simulink model "ACDCMG_woPV"  (R2022a)
settings: Solver=FixedStepAuto  StartTime=0.0  StopTime=0.2  FixedStep=Ts  MaxStep=1e-2  RelTol=1e-3
InitFcn:
  | Set_parameters_R2018
values from neighbouring files (symbols this model uses):
  D_invs = 0.05    [Set_parameters_R2018.m]
  dis11 = 3    [Set_parameters_R2018.m]
  dis14 = 2    [Set_parameters_R2018.m]
  dis2 = 0.2    [Set_parameters_R2018.m]
  dis3 = 0.15    [Set_parameters_R2018.m]
  dis4 = 0.4    [Set_parameters_R2018.m]
  dis5 = 0.4    [Set_parameters_R2018.m]
  dis6 = 0.4    [Set_parameters_R2018.m]
  dis8 = 2    [Set_parameters_R2018.m]
  Fnom = 60    [Set_parameters_R2018.m]
  H_invs = 6    [Set_parameters_R2018.m]
  max_min = 1    [Set_parameters_R2018.m]
  P_Load_3 = S_Load_3* PF_Load_3    (= 25500)    [Set_parameters_R2018.m]
  P_nom_inv = 3e3    (= 3000)    [Set_parameters_R2018.m]
  Pnom_T1 = 1.5e6    (= 1500000)    [Set_parameters_R2018.m]
  Pnom_T2 = 1.5e6    (= 1500000)    [Set_parameters_R2018.m]
  Pnom_T3 = 4e6    (= 4000000)    [Set_parameters_R2018.m]
  Ql_Load_3 = S_Load_3 * sin(acos(PF_Load_3))    [Set_parameters_R2018.m]
  R_Load_9 = (Vnom_prim * 1.35)^2 / P_Load_9    (= 1084.6153125)    [Set_parameters_R2018.m]
  R_Load_DC = Vnom_DC^2/ P_Load_DC    (= 45)    [Set_parameters_R2018.m]
  Rl = 0.394    [Set_parameters_R2018.m]
  Rls = 0.198    [Set_parameters_R2018.m]
  Ts = Ts_Power    (= 6.94444444444e-06)    [Set_parameters_R2018.m]
  Ts_Control = 6*Ts_Power    (= 4.16666666667e-05)    [Set_parameters_R2018.m]
  Ts_Power = 1/(24*Fnom)/100    (= 6.94444444444e-06)    [Set_parameters_R2018.m]
  V1_LL_T3 = 69e3    (= 69000)    [Set_parameters_R2018.m]
  Vnom_DC = 300    [Set_parameters_R2018.m]
  Vnom_Diesel = 2.4e3    (= 2400)    [Set_parameters_R2018.m]
  Vnom_prim = 13.8e3    (= 13800)    [Set_parameters_R2018.m]
  Vnom_sec = 220    [Set_parameters_R2018.m]
  Vnom_ter_AC_DC = 150    [Set_parameters_R2018.m]
  Xl = 0.1168    [Set_parameters_R2018.m]
  Xls = 0.1089    [Set_parameters_R2018.m]
undefined symbols (not defined in the file or in its folder): D1, Delta, DiscIntNeverNeededParam, ee_sli_rtmsupport, fn, gcbh, Ion, Lithium, S, sigbuilder_block, VnInv
libraries: powerlib_extras x55, spsCurrentMeasurementLib x53, powerlib_meascontrol x42, spsSeriesRLCBranchLib x32, spsVoltageMeasurementLib x31, spsRMSLib x29, spsThreePhaseVIMeasurementLib x24, simulink x21, spsThreePhaseSeriesRLCBranchLib x19, spsPower3phInstantaneousLib x15, spsPowerLib x12, spsGroundLib x11
(part 7 of 9)

== system ACDCMG_woPV/Grid Bi-directional Converter 1.2 300 (DC) // 150 V (AC) P_nom 3kW1/Power Measurement (Three-Phase)/Continuous ==
  V : Inport
  I : Inport  Port=2
  Complex to Real-Imag : ComplexToRealImag
  Demux2 : Demux  Outputs=3
  Demux3 : Demux  Outputs=3
  Gain1 : Gain  Gain=3/2
  Gain2 : Gain  Gain=3/2
  Gain3 : Gain  Gain=3/2
  Math Function : Math  Operator=conj  SignedPower=on
  Math Function1 : Math  Operator=conj  SignedPower=on
  Math Function2 : Math  Operator=conj  SignedPower=on
  Multiport Switch : MultiPortSwitch  SaturateOnIntegerOverflow=off  InputSameDT=off
  Mux : Mux  Inputs=3
  Mux1 : Mux  Inputs=3
  Negative I2 : Subsystem
  Negative V2 : Subsystem
  Phase-A I : Subsystem
  Phase-A V : Subsystem
  Phase-B I : Subsystem
  Phase-B V : Subsystem
  Phase-C I : Subsystem
  Phase-C V : Subsystem
  Positive I1 : Subsystem
  Positive V1 : Subsystem
  Product1 : Product
  Product2 : Product
  Product3 : Product
  Sequence : Constant  Value=S
  SinCos : Subsystem
  Zero I0 : Subsystem
  Zero V0 : Subsystem
  P : Outport  VectorParamsAs1DForOutWhenUnconnected=off
  Q : Outport  Port=2  VectorParamsAs1DForOutWhenUnconnected=off
  wires:
  Product3/1 -> Gain2/1
  V/1 -> Demux2/1
  Demux2/1 -> Phase-A V/1(Input)
  Demux2/2 -> Phase-B V/1(Input)
  Demux2/3 -> Phase-C V/1(Input)
  Demux3/3 -> Phase-C I/1(Input)
  Demux3/2 -> Phase-B I/1(Input)
  Demux3/1 -> Phase-A I/1(Input)
  I/1 -> Demux3/1
  SinCos/1(SinCos) -> Phase-C I/2(SinCos), Phase-B I/2(SinCos), Phase-A I/2(SinCos), Phase-C V/2(SinCos), Phase-B V/2(SinCos), Phase-A V/2(SinCos)
  Positive I1/1(I1) -> Math Function/1
  Math Function/1 -> Product3/2
  Phase-A V/1(Phasor) -> Mux/1
  Phase-B V/1(Phasor) -> Mux/2
  Phase-C V/1(Phasor) -> Mux/3
  Mux/1 -> Zero V0/1(Phasor_ABC), Negative V2/1(Phasor_ABC), Positive V1/1(Phasor_ABC)
  Phase-A I/1(Phasor) -> Mux1/1
  Phase-B I/1(Phasor) -> Mux1/2
  Phase-C I/1(Phasor) -> Mux1/3
  Mux1/1 -> Positive I1/1(Phasor_ABC), Negative I2/1(Phasor_ABC), Zero I0/1(Phasor_ABC)
  Positive V1/1(V1) -> Product3/1
  Negative I2/1(I2) -> Math Function1/1
  Zero I0/1(I0) -> Math Function2/1
  Product1/1 -> Gain1/1
  Negative V2/1(V2) -> Product1/1
  Math Function1/1 -> Product1/2
  Product2/1 -> Gain3/1
  Zero V0/1(V0) -> Product2/1
  Math Function2/1 -> Product2/2
  Gain2/1 -> Multiport Switch/2
  Gain1/1 -> Multiport Switch/3
  Gain3/1 -> Multiport Switch/4
  Sequence/1 -> Multiport Switch/1
  Multiport Switch/1 -> Complex to Real-Imag/1
  Complex to Real-Imag/1 -> P/1
  Complex to Real-Imag/2 -> Q/1

== system ACDCMG_woPV/Grid Bi-directional Converter 1.2 300 (DC) // 150 V (AC) P_nom 3kW1/Power Measurement (Three-Phase)/Discrete ==
  V : Inport
  I : Inport  Port=2
  Complex to Real-Imag : ComplexToRealImag
  Demux2 : Demux  Outputs=3
  Demux3 : Demux  Outputs=3
  Gain1 : Gain  Gain=3/2
  Gain2 : Gain  Gain=3/2
  Gain3 : Gain  Gain=3/2
  Math Function : Math  Operator=conj  SignedPower=on
  Math Function1 : Math  Operator=conj  SignedPower=on
  Math Function2 : Math  Operator=conj  SignedPower=on
  Multiport Switch : MultiPortSwitch  SaturateOnIntegerOverflow=off  InputSameDT=off
  Mux : Mux  Inputs=3
  Mux1 : Mux  Inputs=3
  Negative I2 : Subsystem
  Negative V2 : Subsystem
  Phase-A I : Subsystem
  Phase-A V : Subsystem
  Phase-B I : Subsystem
  Phase-B V : Subsystem
  Phase-C I : Subsystem
  Phase-C V : Subsystem
  Positive I1 : Subsystem
  Positive V1 : Subsystem
  Product1 : Product
  Product2 : Product
  Product3 : Product
  Sequence : Constant  Value=S
  SinCos : Subsystem
  Zero I0 : Subsystem
  Zero V0 : Subsystem
  P : Outport  VectorParamsAs1DForOutWhenUnconnected=off
  Q : Outport  Port=2  VectorParamsAs1DForOutWhenUnconnected=off
  wires:
  Complex to Real-Imag/2 -> Q/1
  Complex to Real-Imag/1 -> P/1
  Multiport Switch/1 -> Complex to Real-Imag/1
  Sequence/1 -> Multiport Switch/1
  Gain3/1 -> Multiport Switch/4
  Gain1/1 -> Multiport Switch/3
  Gain2/1 -> Multiport Switch/2
  Math Function2/1 -> Product2/2
  Zero V0/1(V0) -> Product2/1
  Product2/1 -> Gain3/1
  Math Function1/1 -> Product1/2
  Negative V2/1(V2) -> Product1/1
  Product1/1 -> Gain1/1
  Zero I0/1(I0) -> Math Function2/1
  Negative I2/1(I2) -> Math Function1/1
  Positive V1/1(V1) -> Product3/1
  Mux1/1 -> Zero I0/1(Phasor_ABC), Negative I2/1(Phasor_ABC), Positive I1/1(Phasor_ABC)
  Phase-C I/1(Phasor) -> Mux1/3
  Phase-B I/1(Phasor) -> Mux1/2
  Phase-A I/1(Phasor) -> Mux1/1
  Mux/1 -> Positive V1/1(Phasor_ABC), Negative V2/1(Phasor_ABC), Zero V0/1(Phasor_ABC)
  Phase-C V/1(Phasor) -> Mux/3
  Phase-B V/1(Phasor) -> Mux/2
  Phase-A V/1(Phasor) -> Mux/1
  Math Function/1 -> Product3/2
  Positive I1/1(I1) -> Math Function/1
  SinCos/1(SinCos) -> Phase-A V/2(SinCos), Phase-B V/2(SinCos), Phase-C V/2(SinCos), Phase-A I/2(SinCos), Phase-C I/2(SinCos), Phase-B I/2(SinCos)
  I/1 -> Demux3/1
  Demux3/1 -> Phase-A I/1(Input)
  Demux3/2 -> Phase-B I/1(Input)
  Demux3/3 -> Phase-C I/1(Input)
  Demux2/3 -> Phase-C V/1(Input)
  Demux2/2 -> Phase-B V/1(Input)
  Demux2/1 -> Phase-A V/1(Input), SinCos/1(In1)
  V/1 -> Demux2/1
  Product3/1 -> Gain2/1

== system ACDCMG_woPV/Grid Bi-directional Converter 1.2 300 (DC) // 150 V (AC) P_nom 3kW2/Control of Inverter/Discrete PWM Generator1 ==
  note: Pierre Giroux, Gilbert Sybille
      | Power System Laboratory, IREQ
      | Hydro-Quebec
  note: PWM Generator
  Uref : Inport
  BL4 : Logic  Operator=NOT  Inputs=1
  BL5 : Logic  Operator=NOT  Inputs=1
  Constant : Constant  Value=Internal_Phase
  Constant1 : Constant  Value=Internal
  Data Type Conversion : DataTypeConversion  OutDataTypeStr=double
  Data Type Conversion1 : DataTypeConversion  OutDataTypeStr=boolean
  Data Type Conversion2 : DataTypeConversion  OutDataTypeStr=boolean
  Gain : Gain  Gain=2*pi*Freq  SaturateOnIntegerOverflow=on  OutDataTypeStr=Inherit: Same as input  ParamDataTypeStr=Inherit: Same as input
  Gain2 : Gain  Gain=pi/180  SaturateOnIntegerOverflow=on  OutDataTypeStr=Inherit: Same as input  ParamDataTypeStr=Inherit: Same as input
  Gain3 : Gain  Gain=-1  SaturateOnIntegerOverflow=on  OutDataTypeStr=Inherit: Same as input  ParamDataTypeStr=Inherit: Same as input
  Mux : Mux  Inputs=2
  Mux1 : Mux  Inputs=2
  Mux2 : Mux  Inputs=2
  Product : Product  InputSameDT=on  SaturateOnIntegerOverflow=on  OutDataTypeStr=Inherit: Same as first input
  Relational Operator : RelationalOperator
  Relational Operator1 : RelationalOperator
  Select1A : Selector  InputPortWidth=Select1_PortWidth  IndexOptions=Index vector (dialog)  Indices=Select1_Elements  OutputSizes=1
  Select1B : Selector  InputPortWidth=Select1_PortWidth  IndexOptions=Index vector (dialog)  Indices=Select1_Elements  OutputSizes=1
  Select3 : Selector  InputPortWidth=Select3_PortWidth  IndexOptions=Index vector (dialog)  Indices=Select3_Elements  OutputSizes=1
  Sum : Sum  Inputs=+++  InputSameDT=on  SaturateOnIntegerOverflow=on  OutDataTypeStr=Inherit: Same as first input
  Switch : Switch  Criteria=u2 > Threshold  SaturateOnIntegerOverflow=off  InputSameDT=off
  Triangle : simulink/Sources/Repeating Sequence  rep_seq_t=[0 1/Fc/4 3/Fc/4 1/Fc]  rep_seq_y=[0 -1 1 0]
  Trigonometric Function : Trigonometry
  m3 : Constant  Value=Phase
  m4 : Constant  Value=mIndex
  t : DigitalClock  SampleTime=Ts
  Pulses : Outport  VectorParamsAs1DForOutWhenUnconnected=off
  wires:
  Mux2/1 -> Select3/1
  Select1B/1 -> Mux2/2
  Select1A/1 -> Mux2/1
  Mux1/1 -> Select1B/1
  Mux/1 -> Select1A/1
  BL5/1 -> Mux1/2
  BL4/1 -> Mux/2
  Gain3/1 -> Relational Operator1/1
  Triangle/1 -> Relational Operator1/2, Relational Operator/2
  Product/1 -> Switch/1
  Constant1/1 -> Switch/2
  Trigonometric Function/1 -> Product/2
  Sum/1 -> Trigonometric Function/1
  m4/1 -> Product/1
  Constant/1 -> Sum/3
  m3/1 -> Gain2/1
  Gain2/1 -> Sum/2
  Gain/1 -> Sum/1
  t/1 -> Gain/1
  Select3/1 -> Data Type Conversion/1
  Data Type Conversion/1 -> Pulses/1
  Relational Operator/1 -> Data Type Conversion1/1
  Data Type Conversion1/1 -> BL4/1, Mux/1
  Relational Operator1/1 -> Data Type Conversion2/1
  Data Type Conversion2/1 -> BL5/1, Mux1/1
  Switch/1 -> Relational Operator/1, Gain3/1
  Uref/1 -> Switch/3

== system ACDCMG_woPV/Grid Bi-directional Converter 1.2 300 (DC) // 150 V (AC) P_nom 3kW2/Control of Inverter/MI Controller ==
  Vabc : Inport
  DC to AC : Constant  Value=1.2
  Demux : Demux  Commented=on  Outputs=3
  Demux1 : Demux  Outputs=3
  Mux : Mux  Inputs=3
  Mux1 : Mux  Inputs=3
  Mux2 : Mux  Inputs=3
  Product : Product  RndMeth=Zero
  Product1 : Product  RndMeth=Zero
  Product2 : Product  RndMeth=Zero
  Subsystem : Subsystem
  Subsystem1 : Subsystem
  Terminator1 : Terminator  Commented=on
  Terminator2 : Terminator  Commented=on
  Terminator3 : Terminator
  Terminator4 : Terminator
  Terminator5 : Terminator  Commented=on
  Vab1 : powerlib_extras/Discrete Measurements/Discrete  RMS value  Commented=on  Freq=60  Mag_Init=0  Ts=20e-6
      settings: SourceProductBaseCode=PS
  Vab5 : powerlib_extras/Discrete Measurements/Discrete  RMS value  Commented=on  Freq=60  Mag_Init=0  Ts=20e-6
      settings: SourceProductBaseCode=PS
  Vab6 : powerlib_extras/Discrete Measurements/Discrete  RMS value  Commented=on  Freq=60  Mag_Init=0  Ts=20e-6
      settings: SourceProductBaseCode=PS
  Vabc_inv : Outport  VectorParamsAs1DForOutWhenUnconnected=off
  m : Outport  Port=2  VectorParamsAs1DForOutWhenUnconnected=off
  wires:
  Product/1 -> Mux2/1
  Product1/1 -> Mux2/2
  Product2/1 -> Mux2/3
  Mux1/1 -> m/1
  Vabc/1 -> Demux/1
  Demux/1 -> Vab6/1
  Demux/2 -> Vab5/1
  Demux/3 -> Vab1/1
  Demux1/1 -> Product/1, Mux1/1
  Demux1/2 -> Product1/1, Mux1/2
  Demux1/3 -> Product2/1, Mux1/3
  Subsystem/1(Va) -> Product/2
  Subsystem/2(Vb) -> Product1/2
  Subsystem/3(Vc) -> Product2/2
  Mux2/1 -> Vabc_inv/1
  Vab6/1 -> Terminator2/1
  Subsystem1/3(wt) -> Terminator3/1
  Subsystem1/2(sin_cos) -> Subsystem/1(sin_cos)
  Subsystem1/1(Frec) -> Terminator4/1
  DC to AC/1 -> Mux/1, Mux/2, Mux/3
  Mux/1 -> Demux1/1
  Vab5/1 -> Terminator1/1
  Vab1/1 -> Terminator5/1

== system ACDCMG_woPV/Grid Bi-directional Converter 1.2 300 (DC) // 150 V (AC) P_nom 3kW2/Control of Inverter/Positive-Sequence Active & Reactive Power1 ==
  note: Discrete 3-phase Positive-Sequence Active & Reactive Power
  note: Pierre Giroux, Gilbert Sybille
      | Power System Simulation Laboratory
      | IREQ, Hydro-Quebc
  Vabc : Inport  PortDimensions=3
  Iabc : Inport  Port=2  PortDimensions=3
  Deg->Rad : Gain  Gain=pi/180  SaturateOnIntegerOverflow=on  OutDataTypeStr=Inherit: Same as input  ParamDataTypeStr=Inherit: Same as input
  Discrete 3-phase Positive-Sequence Fundamental Value (I) : powerlib_extras/Discrete Measurements/Discrete 3-phase Positive-Sequence Fundamental Value  Freq=Freq  Par_Init=Par_Iinit  Ts=Ts
      settings: SourceProductBaseCode=PS
  Discrete 3-phase Positive-Sequence Fundamental Value (V) : powerlib_extras/Discrete Measurements/Discrete 3-phase Positive-Sequence Fundamental Value  Freq=Freq  Par_Init=Par_Vinit  Ts=Ts
      settings: SourceProductBaseCode=PS
  Gain1 : Gain  Gain=3/2  SaturateOnIntegerOverflow=on  OutDataTypeStr=Inherit: Same as input  ParamDataTypeStr=Inherit: Same as input
  Mag->RMS : Gain  Gain=1/sqrt(2)
  Mux1 : Mux  Inputs=2
  Mux2 : Mux  Inputs=2
  Mux3 : Mux  Inputs=2
  Product : Product  InputSameDT=on  SaturateOnIntegerOverflow=on  OutDataTypeStr=Inherit: Same as first input
  Product1 : Product  InputSameDT=on  SaturateOnIntegerOverflow=on  OutDataTypeStr=Inherit: Same as first input
  Product2 : Product  InputSameDT=on  SaturateOnIntegerOverflow=on  OutDataTypeStr=Inherit: Same as first input
  Sum : Sum  Inputs=+-  InputSameDT=on  SaturateOnIntegerOverflow=on  OutDataTypeStr=Inherit: Same as first input
  Trigonometric Function : Trigonometry
  Trigonometric Function1 : Trigonometry  Operator=cos
  W->kW Var->kvar : Gain  Gain=1/1000
  RMS_V_I : Outport
  P_Q(kW) : Outport  Port=2
  Phase_V_I : Outport  Port=3
  PF : Outport  Port=4
  wires:
  Vabc/1 -> Discrete 3-phase Positive-Sequence Fundamental Value (V)/1
  Iabc/1 -> Discrete 3-phase Positive-Sequence Fundamental Value (I)/1
  Discrete 3-phase Positive-Sequence Fundamental Value (V)/2 -> Sum/1, Mux1/1
  Discrete 3-phase Positive-Sequence Fundamental Value (I)/2 -> Sum/2, Mux1/2
  Sum/1 -> Deg->Rad/1
  Deg->Rad/1 -> Trigonometric Function1/1, Trigonometric Function/1
  Trigonometric Function1/1 -> PF/1, Product/2
  Trigonometric Function/1 -> Product1/1
  Mux2/1 -> Gain1/1
  Product/1 -> Mux2/1
  Product1/1 -> Mux2/2
  Product2/1 -> Product/1, Product1/2
  Discrete 3-phase Positive-Sequence Fundamental Value (V)/1 -> Mux3/1, Product2/1
  Discrete 3-phase Positive-Sequence Fundamental Value (I)/1 -> Mux3/2, Product2/2
  Mux1/1 -> Phase_V_I/1
  Mux3/1 -> Mag->RMS/1
  Mag->RMS/1 -> RMS_V_I/1
  Gain1/1 -> W->kW Var->kvar/1
  W->kW Var->kvar/1 -> P_Q(kW)/1

== system ACDCMG_woPV/Grid Bi-directional Converter 1.2 300 (DC) // 150 V (AC) P_nom 3kW2/Control of Inverter/V//F ==
  e : Inport
  io : Inport  Port=2
  i : Inport  Port=3
  Udc : Inport  Port=4
  Constant : Constant  Value=150*sqrt(2)
  Constant1 : Constant  Value=0
  Subsystem : Subsystem
  UIcontrol : Subsystem
  Pulses : Outport  VectorParamsAs1DForOutWhenUnconnected=off
  wires:
  Constant/1 -> UIcontrol/1(ed_ref)
  Constant1/1 -> UIcontrol/3(eq_ref)
  Udc/1 -> UIcontrol/9(Udc)
  e/1 -> Subsystem/1(e)
  i/1 -> Subsystem/3(i)
  Subsystem/1(ed) -> UIcontrol/2(ed)
  Subsystem/2(eq) -> UIcontrol/4(eq)
  Subsystem/3(iod) -> UIcontrol/5(iod)
  Subsystem/4(ioq) -> UIcontrol/6(ioq)
  Subsystem/8("wt ") -> UIcontrol/8("wt ")
  Subsystem/7(w) -> UIcontrol/7(w)
  Subsystem/5(id) -> UIcontrol/11(id)
  Subsystem/6(iq) -> UIcontrol/10(iq)
  io/1 -> Subsystem/2(io)
  UIcontrol/1(Pulses) -> Pulses/1

== system ACDCMG_woPV/Grid Bi-directional Converter 1.2 300 (DC) // 150 V (AC) P_nom 3kW3/Control of Inverter/Positive-Sequence Active & Reactive Power1 ==
  note: Discrete 3-phase Positive-Sequence Active & Reactive Power
  note: Pierre Giroux, Gilbert Sybille
      | Power System Simulation Laboratory
      | IREQ, Hydro-Quebc
  Vabc : Inport  PortDimensions=3
  Iabc : Inport  Port=2  PortDimensions=3
  Deg->Rad : Gain  Gain=pi/180  SaturateOnIntegerOverflow=on  OutDataTypeStr=Inherit: Same as input  ParamDataTypeStr=Inherit: Same as input
  Discrete 3-phase Positive-Sequence Fundamental Value (I) : powerlib_extras/Discrete Measurements/Discrete 3-phase Positive-Sequence Fundamental Value  Freq=Freq  Par_Init=Par_Iinit  Ts=Ts
      settings: SourceProductBaseCode=PS
  Discrete 3-phase Positive-Sequence Fundamental Value (V) : powerlib_extras/Discrete Measurements/Discrete 3-phase Positive-Sequence Fundamental Value  Freq=Freq  Par_Init=Par_Vinit  Ts=Ts
      settings: SourceProductBaseCode=PS
  Gain1 : Gain  Gain=3/2  SaturateOnIntegerOverflow=on  OutDataTypeStr=Inherit: Same as input  ParamDataTypeStr=Inherit: Same as input
  Mag->RMS : Gain  Gain=1/sqrt(2)
  Mux1 : Mux  Inputs=2
  Mux2 : Mux  Inputs=2
  Mux3 : Mux  Inputs=2
  Product : Product  InputSameDT=on  SaturateOnIntegerOverflow=on  OutDataTypeStr=Inherit: Same as first input
  Product1 : Product  InputSameDT=on  SaturateOnIntegerOverflow=on  OutDataTypeStr=Inherit: Same as first input
  Product2 : Product  InputSameDT=on  SaturateOnIntegerOverflow=on  OutDataTypeStr=Inherit: Same as first input
  Sum : Sum  Inputs=+-  InputSameDT=on  SaturateOnIntegerOverflow=on  OutDataTypeStr=Inherit: Same as first input
  Trigonometric Function : Trigonometry
  Trigonometric Function1 : Trigonometry  Operator=cos
  W->kW Var->kvar : Gain  Gain=1/1000
  RMS_V_I : Outport
  P_Q(kW) : Outport  Port=2
  Phase_V_I : Outport  Port=3
  PF : Outport  Port=4
  wires:
  Vabc/1 -> Discrete 3-phase Positive-Sequence Fundamental Value (V)/1
  Iabc/1 -> Discrete 3-phase Positive-Sequence Fundamental Value (I)/1
  Discrete 3-phase Positive-Sequence Fundamental Value (V)/2 -> Sum/1, Mux1/1
  Discrete 3-phase Positive-Sequence Fundamental Value (I)/2 -> Sum/2, Mux1/2
  Sum/1 -> Deg->Rad/1
  Deg->Rad/1 -> Trigonometric Function1/1, Trigonometric Function/1
  Trigonometric Function1/1 -> PF/1, Product/2
  Trigonometric Function/1 -> Product1/1
  Mux2/1 -> Gain1/1
  Product/1 -> Mux2/1
  Product1/1 -> Mux2/2
  Product2/1 -> Product/1, Product1/2
  Discrete 3-phase Positive-Sequence Fundamental Value (V)/1 -> Mux3/1, Product2/1
  Discrete 3-phase Positive-Sequence Fundamental Value (I)/1 -> Mux3/2, Product2/2
  Mux1/1 -> Phase_V_I/1
  Mux3/1 -> Mag->RMS/1
  Mag->RMS/1 -> RMS_V_I/1
  Gain1/1 -> W->kW Var->kvar/1
  W->kW Var->kvar/1 -> P_Q(kW)/1

== system ACDCMG_woPV/Grid Bi-directional Converter 1.2 300 (DC) // 150 V (AC) P_nom 3kW3/Control of Inverter/V//F ==
  e : Inport
  io : Inport  Port=2
  i : Inport  Port=3
  Udc : Inport  Port=4
  Constant : Constant  Value=150*sqrt(2)
  Constant1 : Constant  Value=0
  Constant2 : Constant  Commented=on
  Constant3 : Constant  Commented=on
  Constant4 : Constant
  From : From  Commented=on  GotoTag=P_mea_inv  TagVisibility=global
  Gain : Gain  Commented=on  Gain=1/P_nom_inv
  Gain1 : Gain  Gain=Fnom
  Gain2 : Gain  Commented=on  Gain=-1
  Scope : Scope  NumInputPorts=2
  Subsystem : Subsystem
  Sum : Sum  Commented=on  Inputs=|+-
  Sum1 : Sum  Commented=on  Inputs=|++
  Transfer Fcn : TransferFcn  Commented=on  Denominator=[2*H_invs D_invs]
  UIcontrol : Subsystem
  wires:
  Constant/1 -> UIcontrol/1(ed_ref)
  Constant1/1 -> UIcontrol/3(eq_ref)
  Udc/1 -> UIcontrol/9(Udc)
  e/1 -> Subsystem/1(e)
  i/1 -> Subsystem/3(i)
  Subsystem/1(ed) -> UIcontrol/2(ed)
  Subsystem/2(eq) -> UIcontrol/4(eq)
  Subsystem/3(iod) -> UIcontrol/5(iod)
  Subsystem/4(ioq) -> UIcontrol/6(ioq)
  Subsystem/8("wt ") -> UIcontrol/8("wt ")
  Subsystem/7(w) -> UIcontrol/7(w)
  Subsystem/5(id) -> UIcontrol/11(id)
  Subsystem/6(iq) -> UIcontrol/10(iq)
  io/1 -> Subsystem/2(io)
  From/1 -> Gain/1
  Gain1/1 -> Scope/1, Subsystem/4(fcmd)
  Gain/1 -> Scope/2, Sum/1
  Constant2/1 -> Sum/2
  Sum/1 -> Gain2/1
  Gain2/1 -> Transfer Fcn/1
  Transfer Fcn/1 -> Sum1/1
  Constant3/1 -> Sum1/2
  Constant4/1 -> Gain1/1

== system ACDCMG_woPV/Inverter 300 (DC) // 150 V (AC) P_nom 3kW4/Control of Inverter/Positive-Sequence Active & Reactive Power1 ==
  note: Discrete 3-phase Positive-Sequence Active & Reactive Power
  note: Pierre Giroux, Gilbert Sybille
      | Power System Simulation Laboratory
      | IREQ, Hydro-Quebc
  Vabc : Inport  PortDimensions=3
  Iabc : Inport  Port=2  PortDimensions=3
  Deg->Rad : Gain  Gain=pi/180  SaturateOnIntegerOverflow=on  OutDataTypeStr=Inherit: Same as input  ParamDataTypeStr=Inherit: Same as input
  Discrete 3-phase Positive-Sequence Fundamental Value (I) : powerlib_extras/Discrete Measurements/Discrete 3-phase Positive-Sequence Fundamental Value  Freq=Freq  Par_Init=Par_Iinit  Ts=Ts
      settings: SourceProductBaseCode=PS
  Discrete 3-phase Positive-Sequence Fundamental Value (V) : powerlib_extras/Discrete Measurements/Discrete 3-phase Positive-Sequence Fundamental Value  Freq=Freq  Par_Init=Par_Vinit  Ts=Ts
      settings: SourceProductBaseCode=PS
  Gain1 : Gain  Gain=3/2  SaturateOnIntegerOverflow=on  OutDataTypeStr=Inherit: Same as input  ParamDataTypeStr=Inherit: Same as input
  Mag->RMS : Gain  Gain=1/sqrt(2)
  Mux1 : Mux  Inputs=2
  Mux2 : Mux  Inputs=2
  Mux3 : Mux  Inputs=2
  Product : Product  InputSameDT=on  SaturateOnIntegerOverflow=on  OutDataTypeStr=Inherit: Same as first input
  Product1 : Product  InputSameDT=on  SaturateOnIntegerOverflow=on  OutDataTypeStr=Inherit: Same as first input
  Product2 : Product  InputSameDT=on  SaturateOnIntegerOverflow=on  OutDataTypeStr=Inherit: Same as first input
  Sum : Sum  Inputs=+-  InputSameDT=on  SaturateOnIntegerOverflow=on  OutDataTypeStr=Inherit: Same as first input
  Trigonometric Function : Trigonometry
  Trigonometric Function1 : Trigonometry  Operator=cos
  W->kW Var->kvar : Gain  Gain=1/1000
  RMS_V_I : Outport
  P_Q(kW) : Outport  Port=2
  Phase_V_I : Outport  Port=3
  PF : Outport  Port=4
  wires:
  Vabc/1 -> Discrete 3-phase Positive-Sequence Fundamental Value (V)/1
  Iabc/1 -> Discrete 3-phase Positive-Sequence Fundamental Value (I)/1
  Discrete 3-phase Positive-Sequence Fundamental Value (V)/2 -> Sum/1, Mux1/1
  Discrete 3-phase Positive-Sequence Fundamental Value (I)/2 -> Sum/2, Mux1/2
  Sum/1 -> Deg->Rad/1
  Deg->Rad/1 -> Trigonometric Function1/1, Trigonometric Function/1
  Trigonometric Function1/1 -> PF/1, Product/2
  Trigonometric Function/1 -> Product1/1
  Mux2/1 -> Gain1/1
  Product/1 -> Mux2/1
  Product1/1 -> Mux2/2
  Product2/1 -> Product/1, Product1/2
  Discrete 3-phase Positive-Sequence Fundamental Value (V)/1 -> Mux3/1, Product2/1
  Discrete 3-phase Positive-Sequence Fundamental Value (I)/1 -> Mux3/2, Product2/2
  Mux1/1 -> Phase_V_I/1
  Mux3/1 -> Mag->RMS/1
  Mag->RMS/1 -> RMS_V_I/1
  Gain1/1 -> W->kW Var->kvar/1
  W->kW Var->kvar/1 -> P_Q(kW)/1

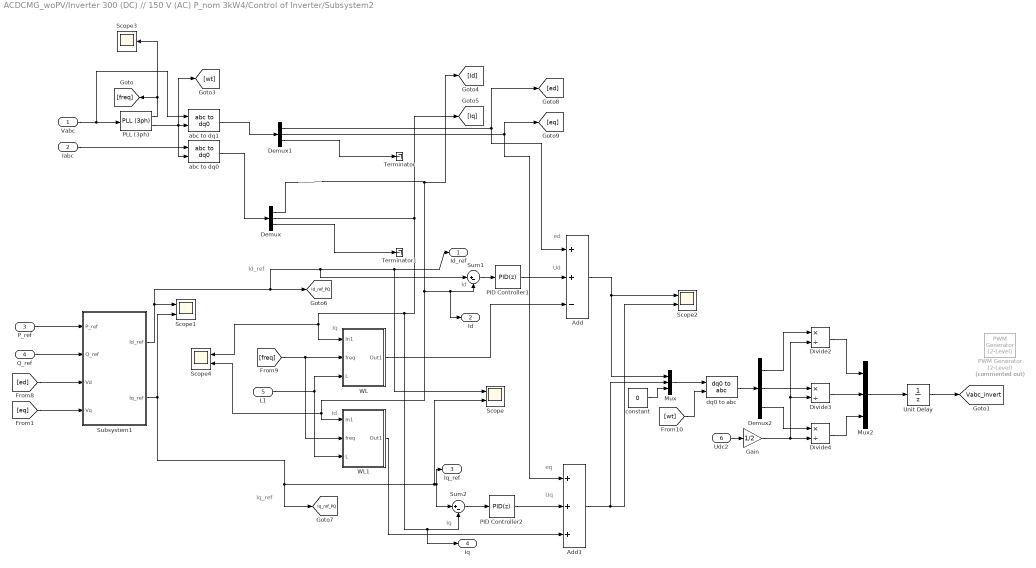
== system ACDCMG_woPV/Inverter 300 (DC) // 150 V (AC) P_nom 3kW4/Control of Inverter/Subsystem2 ==
  note: Iq_ref
  note: Id
  note: Id_ref
  note: Ud
  note: Uq
  note: eq
  note: ed
  note: Iq
  note: Id
  note: Iq
  Vabc : Inport
  Iabc : Inport  Port=2
  P_ref : Inport  Port=3
  Q_ref : Inport  Port=4
  L1 : Inport  Port=5
  Udc2 : Inport  Port=6
  Add : Sum  Inputs=++-
  Add1 : Sum  Inputs=+++
  Demux : Demux  Outputs=3
  Demux1 : Demux  Outputs=3
  Demux2 : Demux  Outputs=3
  Divide2 : Product  Inputs=*/
  Divide3 : Product  Inputs=*/
  Divide4 : Product  Inputs=*/
  Gain : Gain  Gain=1/2
  Mux : Mux  Inputs=3
  Mux2 : Mux  Inputs=3
  PID Controller1 : slpidlib/PID Controller  Controller=PID  Form=Parallel  TimeDomain=Discrete-time  UseExternalTs=off  SampleTime=Ts_Control  IntegratorMethod=Forward Euler  FilterMethod=Forward Euler  ControllerParametersSource=internal  P=Kp  I=Ki  UseKiTs=off  D=Kd  N=100  UseFilter=on  TunerSelectOption=Transfer Function Based (PID Tuner App)  InitialConditionSource=internal  InitialConditionForIntegrator=0  InitialConditionForFilter=0  DifferentiatorICPrevScaledInput=0  ExternalReset=none  TrackingMode=off  Kt=1  LimitOutput=off  SatLimitsSource=internal  UpperSaturationLimit=inf  LowerSaturationLimit=-inf  LinearizeAsGain=on  AntiWindupMode=none  Kb=1  POutMin=[]  POutMax=[]  IOutMin=[]  IOutMax=[]  DOutMin=[]  DOutMax=[]  NOutMin=[]  NOutMax=[]  SumOutMin=[]  SumOutMax=[]  SaturationOutMin=[]  SaturationOutMax=[]  PParamMin=[]  PParamMax=[]  IParamMin=[]  IParamMax=[]  DParamMin=[]  DParamMax=[]  NParamMin=[]  NParamMax=[]  KbParamMin=[]  KbParamMax=[]  KtParamMin=[]  KtParamMax=[]  KbOutMin=[]  KbOutMax=[]  KtOutMin=[]  KtOutMax=[]  IntegratorOutMin=[]  IntegratorOutMax=[]  FilterOutMin=[]  FilterOutMax=[]  SumI1OutMin=[]  SumI1OutMax=[]  SumI2OutMin=[]  SumI2OutMax=[]  SumI3OutMin=[]  SumI3OutMax=[]  SumI4OutMin=[]  SumI4OutMax=[]  SumDOutMin=[]  SumDOutMax=[]  DifferentiatorOutMin=[]  DifferentiatorOutMax=[]  FilterDiffOutCoefMin=[]  FilterDiffOutCoefMax=[]  ReciprocalOutMin=[]  ReciprocalOutMax=[]  SumDenOutMin=[]  SumDenOutMax=[]  SumNumOutMin=[]  SumNumOutMax=[]  DivideOutMin=[]  DivideOutMax=[]  UdiffTsProdOutMin=[]  UdiffTsProdOutMax=[]  NTsProdOutMin=[]  NTsProdOutMax=[]  UintegralTsProdOutMin=[]  UintegralTsProdOutMax=[]  UngainTsProdOutMin=[]  UngainTsProdOutMax=[]  IntegratorContinuousStateAttributes=''  IntegratorStateMustResolveToSignalObject=off  IntegratorRTWStateStorageClass=Auto  FilterContinuousStateAttributes=''  FilterStateMustResolveToSignalObject=off  FilterRTWStateStorageClass=Auto  ParallelPVariant=InternalParameters  IdealPVariant=Disabled  IVariant=InternalParameters  DVariant=InternalParameters  IntegratorVariant=Discrete  SatVariant=Disabled  AWVariant=Passthrough  PCopyVariant=Disabled  TRVariant=Disabled  FdbkBlocksVariant=Forward  IdealPFdbkVariant=Disabled  SatFdbkVariant=Disabled  DerivativeFilterVariant=ForwardEulerFilter  NVariant=InternalParameters  NCopyVariant=Disabled  FilterICVariant=InternalICsFilter  IntegratorICVariant=InternalICs  ExternalResetVariant=Disabled  TRSumVariant=Passthrough  SumFdbkVariant=Disabled  SumVariant=Sum_PID  TsampFilterVariant=InternalTs  TsampNgainVariant=Passthrough  TsampIntegralVariant=Passthrough  ExternalSaturationOutDataTypeStr=Inherit: Same as second input  aMode=0
  PID Controller2 : slpidlib/PID Controller  Controller=PID  Form=Parallel  TimeDomain=Discrete-time  UseExternalTs=off  SampleTime=Ts_Control  IntegratorMethod=Forward Euler  FilterMethod=Forward Euler  ControllerParametersSource=internal  P=Kp  I=Ki  UseKiTs=off  D=Kd  N=100  UseFilter=on  TunerSelectOption=Transfer Function Based (PID Tuner App)  InitialConditionSource=internal  InitialConditionForIntegrator=0  InitialConditionForFilter=0  DifferentiatorICPrevScaledInput=0  ExternalReset=none  TrackingMode=off  Kt=1  LimitOutput=off  SatLimitsSource=internal  UpperSaturationLimit=inf  LowerSaturationLimit=-inf  LinearizeAsGain=on  AntiWindupMode=none  Kb=1  POutMin=[]  POutMax=[]  IOutMin=[]  IOutMax=[]  DOutMin=[]  DOutMax=[]  NOutMin=[]  NOutMax=[]  SumOutMin=[]  SumOutMax=[]  SaturationOutMin=[]  SaturationOutMax=[]  PParamMin=[]  PParamMax=[]  IParamMin=[]  IParamMax=[]  DParamMin=[]  DParamMax=[]  NParamMin=[]  NParamMax=[]  KbParamMin=[]  KbParamMax=[]  KtParamMin=[]  KtParamMax=[]  KbOutMin=[]  KbOutMax=[]  KtOutMin=[]  KtOutMax=[]  IntegratorOutMin=[]  IntegratorOutMax=[]  FilterOutMin=[]  FilterOutMax=[]  SumI1OutMin=[]  SumI1OutMax=[]  SumI2OutMin=[]  SumI2OutMax=[]  SumI3OutMin=[]  SumI3OutMax=[]  SumI4OutMin=[]  SumI4OutMax=[]  SumDOutMin=[]  SumDOutMax=[]  DifferentiatorOutMin=[]  DifferentiatorOutMax=[]  FilterDiffOutCoefMin=[]  FilterDiffOutCoefMax=[]  ReciprocalOutMin=[]  ReciprocalOutMax=[]  SumDenOutMin=[]  SumDenOutMax=[]  SumNumOutMin=[]  SumNumOutMax=[]  DivideOutMin=[]  DivideOutMax=[]  UdiffTsProdOutMin=[]  UdiffTsProdOutMax=[]  NTsProdOutMin=[]  NTsProdOutMax=[]  UintegralTsProdOutMin=[]  UintegralTsProdOutMax=[]  UngainTsProdOutMin=[]  UngainTsProdOutMax=[]  IntegratorContinuousStateAttributes=''  IntegratorStateMustResolveToSignalObject=off  IntegratorRTWStateStorageClass=Auto  FilterContinuousStateAttributes=''  FilterStateMustResolveToSignalObject=off  FilterRTWStateStorageClass=Auto  ParallelPVariant=InternalParameters  IdealPVariant=Disabled  IVariant=InternalParameters  DVariant=InternalParameters  IntegratorVariant=Discrete  SatVariant=Disabled  AWVariant=Passthrough  PCopyVariant=Disabled  TRVariant=Disabled  FdbkBlocksVariant=Forward  IdealPFdbkVariant=Disabled  SatFdbkVariant=Disabled  DerivativeFilterVariant=ForwardEulerFilter  NVariant=InternalParameters  NCopyVariant=Disabled  FilterICVariant=InternalICsFilter  IntegratorICVariant=InternalICs  ExternalResetVariant=Disabled  TRSumVariant=Passthrough  SumFdbkVariant=Disabled  SumVariant=Sum_PID  TsampFilterVariant=InternalTs  TsampNgainVariant=Passthrough  TsampIntegralVariant=Passthrough  ExternalSaturationOutDataTypeStr=Inherit: Same as second input  aMode=0
  PLL (3ph) : spsPLL3phLib/PLL (3ph)  Fmin=59.5  Par_Init=[0, 60]  ParK=[180, 3200, 1]  TcD=1e-4  MaxRateChangeFreq=12  FilterCutOffFreq=25  Ts=Ts_Control  AGC=on
  PWM Generator (2-Level) : spsPWMGenerator2LevelLib/PWM Generator (2-Level)  Commented=on  ModulatorType=Three-phase bridge (6 pulses)  ModulatorMode=Unsynchronized  Fc=15000  Pc=90  nF=27  MinMax="[ -1  1 ]"  SamplingTechnique=Natural  ModulatingSignals=off  m=0.8  Freq=60  Phase=0  Ts=Ts_Power  ShowCarrierOutport=off
  Scope{,1..2,4} (4 alike) : Scope  NumInputPorts=2
  Scope3 : Scope
  Subsystem1 : Subsystem
  Sum1 : Sum  Inputs=|+-
  Sum2 : Sum  Inputs=|+-
  Terminator : Terminator
  Terminator1 : Terminator
  Unit Delay : UnitDelay  SampleTime=-1  HasFrameUpgradeWarning=on
  WL : Subsystem
  WL1 : Subsystem
  abc to dq0 : spsabctodq0Lib/abc to dq0  Alignment=90 degrees behind phase A axis
  abc to dq1 : spsabctodq0Lib/abc to dq0  Alignment=90 degrees behind phase A axis
  constant : Constant  Value=0
  dq0 to abc : spsdq0toabcLib/dq0 to abc  Alignment=90 degrees behind phase A axis
  Id_ref : Outport
  Id : Outport  Port=2
  Iq_ref : Outport  Port=3
  Iq : Outport  Port=4
  tag scope: Id_ref_PQ=global, Iq_ref_PQ=global, Vabc_invert=global
  wires:
  abc to dq1/1 -> Demux1/1
  Sum1/1 -> PID Controller1/1
  Iabc/1 -> abc to dq0/1
  Vabc/1 -> abc to dq1/1, PLL (3ph)/1
  PLL (3ph)/2 -> [wt], abc to dq1/2, abc to dq0/2
  Demux1/1 -> Add/1, [ed]
  L1/1 -> WL/3(L), WL1/3(L)
  WL/1(Out1) -> Add/3
  [freq] -> WL1/2(freq), WL/2(freq)
  PLL (3ph)/1 -> Scope3/1, [freq]
  Demux2/1 -> Divide2/1
  Add/1 -> Mux/1, Scope2/1
  PID Controller2/1 -> Add1/2
  Sum2/1 -> PID Controller2/1
  Demux2/2 -> Divide3/1
  WL1/1(Out1) -> Add1/3
  Demux1/2 -> Add1/1, [eq]
  Add1/1 -> Mux/2, Scope2/2
  Gain/1 -> Divide3/2, Divide2/2, Divide4/2
  Divide4/1 -> Mux2/3
  Divide2/1 -> Mux2/1
  Mux/1 -> dq0 to abc/1
  Demux2/3 -> Divide4/1
  Divide3/1 -> Mux2/2
  dq0 to abc/1 -> Demux2/1
  PID Controller1/1 -> Add/2
  [wt] -> dq0 to abc/2
  Udc2/1 -> Gain/1
  Demux1/3 -> Terminator/1
  Demux/3 -> Terminator1/1
  constant/1 -> Mux/3
  P_ref/1 -> Subsystem1/1(P_ref)
  Q_ref/1 -> Subsystem1/2(Q_ref)
  [ed] -> Subsystem1/3(Vd)
  [eq] -> Subsystem1/4(Vq)
  Subsystem1/2(Iq_ref) -> Scope1/2, [Iq_ref_PQ], Scope/2, Iq_ref/1, Sum2/1
  Subsystem1/1(Id_ref) -> Sum1/1, Scope/1, Id_ref/1, [Id_ref_PQ], Scope1/1
  Demux/1 -> Scope4/2, WL1/1(In1), Id/1, Sum1/2, [Id]
  Demux/2 -> [Iq], Scope4/1, WL/1(In1), Iq/1, Sum2/2
  abc to dq0/1 -> Demux/1
  Mux2/1 -> Unit Delay/1
  Unit Delay/1 -> [Vabc_invert]

== system ACDCMG_woPV/Inverter 300 (DC) // 150 V (AC) P_nom 3kW4/Control of Inverter/V//F ==
  e : Inport
  io : Inport  Port=2
  i : Inport  Port=3
  Udc : Inport  Port=4
  Constant : Constant  Value=150*sqrt(2)
  Constant1 : Constant  Value=0
  Constant2 : Constant  Commented=on
  Constant3 : Constant  Commented=on
  Constant4 : Constant
  From : From  Commented=on  GotoTag=P_mea_inv  TagVisibility=global
  Gain : Gain  Commented=on  Gain=1/P_nom_inv
  Gain1 : Gain  Gain=Fnom
  Gain2 : Gain  Commented=on  Gain=-1
  Scope : Scope  NumInputPorts=2
  Subsystem : Subsystem
  Sum : Sum  Commented=on  Inputs=|+-
  Sum1 : Sum  Commented=on  Inputs=|++
  Transfer Fcn : TransferFcn  Commented=on  Denominator=[2*H_invs D_invs]
  UIcontrol : Subsystem
  wires:
  Constant/1 -> UIcontrol/1(ed_ref)
  Constant1/1 -> UIcontrol/3(eq_ref)
  Udc/1 -> UIcontrol/9(Udc)
  e/1 -> Subsystem/1(e)
  i/1 -> Subsystem/3(i)
  Subsystem/1(ed) -> UIcontrol/2(ed)
  Subsystem/2(eq) -> UIcontrol/4(eq)
  Subsystem/3(iod) -> UIcontrol/5(iod)
  Subsystem/4(ioq) -> UIcontrol/6(ioq)
  Subsystem/8("wt ") -> UIcontrol/8("wt ")
  Subsystem/7(w) -> UIcontrol/7(w)
  Subsystem/5(id) -> UIcontrol/11(id)
  Subsystem/6(iq) -> UIcontrol/10(iq)
  io/1 -> Subsystem/2(io)
  From/1 -> Gain/1
  Gain1/1 -> Scope/1, Subsystem/4(fcmd)
  Gain/1 -> Scope/2, Sum/1
  Constant2/1 -> Sum/2
  Sum/1 -> Gain2/1
  Gain2/1 -> Transfer Fcn/1
  Transfer Fcn/1 -> Sum1/1
  Constant3/1 -> Sum1/2
  Constant4/1 -> Gain1/1

== system ACDCMG_woPV/Grid Bi-directional Converter 1.1 300 (DC) // 150 V (AC) P_nom 3kW/Control of Inverter/MI Controller/OP max // min ==
  note: DC to AC
  note: AC to DC
  Constant2 : Constant  Value=max_min
  OP_max1 : Constant  Value=1.2
  OP_min1 : Constant
  Switch2 : Switch  Criteria=u2 > Threshold  SaturateOnIntegerOverflow=off  InputSameDT=off
  ctrl : Outport  VectorParamsAs1DForOutWhenUnconnected=off
  wires:
  OP_max1/1 -> Switch2/1
  OP_min1/1 -> Switch2/3
  Constant2/1 -> Switch2/2
  Switch2/1 -> ctrl/1

== system ACDCMG_woPV/Grid Bi-directional Converter 1.1 300 (DC) // 150 V (AC) P_nom 3kW/Control of Inverter/MI Controller/Subsystem ==
  sin_cos : Inport  PortDimensions=2
  Demux : Demux  Outputs=2
      settings: DisplayOption=none
  Fcn2 : Fcn  Expr=1*u[1]
  Fcn4 : Fcn  Expr=1*u[3]
  Fcn5 : Fcn  Expr=1*u[5]
  K1 : Constant  Value=0.5
  K2 : Constant  Value=sqrt(3)/2
  Mux2 : Mux  Inputs=6
  Product{,1..3} (4 alike) : Product  InputSameDT=on  SaturateOnIntegerOverflow=on  OutDataTypeStr=Inherit: Same as first input
  Sum : Sum  Inputs=--  InputSameDT=on  SaturateOnIntegerOverflow=on  OutDataTypeStr=Inherit: Same as first input
  Sum1 : Sum  Inputs=-+  InputSameDT=on  SaturateOnIntegerOverflow=on  OutDataTypeStr=Inherit: Same as first input
  Sum2 : Sum  Inputs=--  InputSameDT=on  SaturateOnIntegerOverflow=on  OutDataTypeStr=Inherit: Same as first input
  Sum3 : Sum  Inputs=--  InputSameDT=on  SaturateOnIntegerOverflow=on  OutDataTypeStr=Inherit: Same as first input
  Va : Outport  VectorParamsAs1DForOutWhenUnconnected=off
  Vb : Outport  Port=2  VectorParamsAs1DForOutWhenUnconnected=off
  Vc : Outport  Port=3  VectorParamsAs1DForOutWhenUnconnected=off
  wires:
  sin_cos/1 -> Demux/1
  Demux/1 -> Product/1, Product2/1, Sum2/2, Mux2/1  "sin(wt)"
  Product/1 -> Sum/1
  Product1/1 -> Sum/2
  Product3/1 -> Sum1/1
  Product2/1 -> Sum1/2
  Sum3/1 -> Mux2/6  "cos(wt+2pi/3)"
  Sum2/1 -> Mux2/5  "sin(wt+2pi/3)"
  K1/1 -> Product/2, Product3/2
  K2/1 -> Product1/2, Product2/2
  Sum/1 -> Mux2/3, Sum2/1  "sin(wt-2pi/3)"
  Sum1/1 -> Mux2/4, Sum3/1  "cos(wt-2pi/3)"
  Demux/2 -> Sum3/2, Product3/1, Product1/1, Mux2/2  "cos(wt)"
  Mux2/1 -> Fcn2/1, Fcn4/1, Fcn5/1
  Fcn2/1 -> Va/1
  Fcn4/1 -> Vb/1
  Fcn5/1 -> Vc/1

== system ACDCMG_woPV/Grid Bi-directional Converter 1.1 300 (DC) // 150 V (AC) P_nom 3kW/Control of Inverter/MI Controller/Subsystem1 ==
  note: AC to DC
  note: DC to AC
  Constant1 : Constant  Value=max_min
  Constant2 : Constant  Value=2*pi
  Deg->Rad : Gain  Gain=pi/180  SaturateOnIntegerOverflow=on  OutDataTypeStr=Inherit: Same as input  ParamDataTypeStr=Inherit: Same as input
  Freq1 : Constant  Value=Fnom
  Freq2 : Constant  Value=2*pi
  Math Function : Math  Operator=mod  SignedPower=on
  Mux5 : Mux  Inputs=2
  OP_max1 : Constant  Value=0
  OP_min1 : Constant  Value=228
  Product7 : Product  Inputs=***  InputSameDT=on  SaturateOnIntegerOverflow=on  OutDataTypeStr=Inherit: Same as first input
  Sum : Sum  InputSameDT=on  SaturateOnIntegerOverflow=on  OutDataTypeStr=Inherit: Same as first input
  Switch2 : Switch  Criteria=u2 > Threshold  SaturateOnIntegerOverflow=off  InputSameDT=off
  Trigonometric Function : Trigonometry
  Trigonometric Function1 : Trigonometry  Operator=cos
  t : DigitalClock  SampleTime=Ts
  Frec : Outport  VectorParamsAs1DForOutWhenUnconnected=off
  sin_cos : Outport  Port=2  VectorParamsAs1DForOutWhenUnconnected=off
  wt : Outport  Port=3  VectorParamsAs1DForOutWhenUnconnected=off
  wires:
  Switch2/1 -> Deg->Rad/1
  Deg->Rad/1 -> Sum/2
  Freq1/1 -> Frec/1, Product7/1
  Trigonometric Function/1 -> Mux5/1
  Sum/1 -> Math Function/1
  Trigonometric Function1/1 -> Mux5/2
  Product7/1 -> Sum/1
  Freq2/1 -> Product7/3
  Constant2/1 -> Math Function/2
  t/1 -> Product7/2
  Math Function/1 -> wt/1, Trigonometric Function1/1, Trigonometric Function/1
  Mux5/1 -> sin_cos/1
  Constant1/1 -> Switch2/2
  OP_max1/1 -> Switch2/1
  OP_min1/1 -> Switch2/3

== system ACDCMG_woPV/Grid Bi-directional Converter 1.1 300 (DC) // 150 V (AC) P_nom 3kW1/Control of Inverter/MI Controller/OP max // min ==
  note: DC to AC
  note: AC to DC
  Constant2 : Constant  Value=max_min
  OP_max1 : Constant  Value=1.2
  OP_min1 : Constant
  Switch2 : Switch  Criteria=u2 > Threshold  SaturateOnIntegerOverflow=off  InputSameDT=off
  ctrl : Outport  VectorParamsAs1DForOutWhenUnconnected=off
  wires:
  OP_max1/1 -> Switch2/1
  OP_min1/1 -> Switch2/3
  Constant2/1 -> Switch2/2
  Switch2/1 -> ctrl/1

== system ACDCMG_woPV/Grid Bi-directional Converter 1.1 300 (DC) // 150 V (AC) P_nom 3kW1/Control of Inverter/MI Controller/Subsystem ==
  sin_cos : Inport  PortDimensions=2
  Demux : Demux  Outputs=2
      settings: DisplayOption=none
  Fcn2 : Fcn  Expr=1*u[1]
  Fcn4 : Fcn  Expr=1*u[3]
  Fcn5 : Fcn  Expr=1*u[5]
  K1 : Constant  Value=0.5
  K2 : Constant  Value=sqrt(3)/2
  Mux2 : Mux  Inputs=6
  Product{,1..3} (4 alike) : Product  InputSameDT=on  SaturateOnIntegerOverflow=on  OutDataTypeStr=Inherit: Same as first input
  Sum : Sum  Inputs=--  InputSameDT=on  SaturateOnIntegerOverflow=on  OutDataTypeStr=Inherit: Same as first input
  Sum1 : Sum  Inputs=-+  InputSameDT=on  SaturateOnIntegerOverflow=on  OutDataTypeStr=Inherit: Same as first input
  Sum2 : Sum  Inputs=--  InputSameDT=on  SaturateOnIntegerOverflow=on  OutDataTypeStr=Inherit: Same as first input
  Sum3 : Sum  Inputs=--  InputSameDT=on  SaturateOnIntegerOverflow=on  OutDataTypeStr=Inherit: Same as first input
  Va : Outport  VectorParamsAs1DForOutWhenUnconnected=off
  Vb : Outport  Port=2  VectorParamsAs1DForOutWhenUnconnected=off
  Vc : Outport  Port=3  VectorParamsAs1DForOutWhenUnconnected=off
  wires:
  sin_cos/1 -> Demux/1
  Demux/1 -> Product/1, Product2/1, Sum2/2, Mux2/1  "sin(wt)"
  Product/1 -> Sum/1
  Product1/1 -> Sum/2
  Product3/1 -> Sum1/1
  Product2/1 -> Sum1/2
  Sum3/1 -> Mux2/6  "cos(wt+2pi/3)"
  Sum2/1 -> Mux2/5  "sin(wt+2pi/3)"
  K1/1 -> Product/2, Product3/2
  K2/1 -> Product1/2, Product2/2
  Sum/1 -> Mux2/3, Sum2/1  "sin(wt-2pi/3)"
  Sum1/1 -> Mux2/4, Sum3/1  "cos(wt-2pi/3)"
  Demux/2 -> Sum3/2, Product3/1, Product1/1, Mux2/2  "cos(wt)"
  Mux2/1 -> Fcn2/1, Fcn4/1, Fcn5/1
  Fcn2/1 -> Va/1
  Fcn4/1 -> Vb/1
  Fcn5/1 -> Vc/1

== system ACDCMG_woPV/Grid Bi-directional Converter 1.1 300 (DC) // 150 V (AC) P_nom 3kW1/Control of Inverter/MI Controller/Subsystem1 ==
  note: AC to DC
  note: DC to AC
  Constant1 : Constant  Value=max_min
  Constant2 : Constant  Value=2*pi
  Deg->Rad : Gain  Gain=pi/180  SaturateOnIntegerOverflow=on  OutDataTypeStr=Inherit: Same as input  ParamDataTypeStr=Inherit: Same as input
  Freq1 : Constant  Value=Fnom
  Freq2 : Constant  Value=2*pi
  Math Function : Math  Operator=mod  SignedPower=on
  Mux5 : Mux  Inputs=2
  OP_max1 : Constant  Value=0
  OP_min1 : Constant  Value=228
  Product7 : Product  Inputs=***  InputSameDT=on  SaturateOnIntegerOverflow=on  OutDataTypeStr=Inherit: Same as first input
  Sum : Sum  InputSameDT=on  SaturateOnIntegerOverflow=on  OutDataTypeStr=Inherit: Same as first input
  Switch2 : Switch  Criteria=u2 > Threshold  SaturateOnIntegerOverflow=off  InputSameDT=off
  Trigonometric Function : Trigonometry
  Trigonometric Function1 : Trigonometry  Operator=cos
  t : DigitalClock  SampleTime=Ts
  Frec : Outport  VectorParamsAs1DForOutWhenUnconnected=off
  sin_cos : Outport  Port=2  VectorParamsAs1DForOutWhenUnconnected=off
  wt : Outport  Port=3  VectorParamsAs1DForOutWhenUnconnected=off
  wires:
  Switch2/1 -> Deg->Rad/1
  Deg->Rad/1 -> Sum/2
  Freq1/1 -> Frec/1, Product7/1
  Trigonometric Function/1 -> Mux5/1
  Sum/1 -> Math Function/1
  Trigonometric Function1/1 -> Mux5/2
  Product7/1 -> Sum/1
  Freq2/1 -> Product7/3
  Constant2/1 -> Math Function/2
  t/1 -> Product7/2
  Math Function/1 -> wt/1, Trigonometric Function1/1, Trigonometric Function/1
  Mux5/1 -> sin_cos/1
  Constant1/1 -> Switch2/2
  OP_max1/1 -> Switch2/1
  OP_min1/1 -> Switch2/3

== system ACDCMG_woPV/Grid Bi-directional Converter 1.1 300 (DC) // 150 V (AC) P_nom 3kW2/Control of Inverter/MI Controller/OP max // min ==
  note: DC to AC
  note: AC to DC
  Constant2 : Constant  Value=max_min
  OP_max1 : Constant  Value=1.2
  OP_min1 : Constant
  Switch2 : Switch  Criteria=u2 > Threshold  SaturateOnIntegerOverflow=off  InputSameDT=off
  ctrl : Outport  VectorParamsAs1DForOutWhenUnconnected=off
  wires:
  OP_max1/1 -> Switch2/1
  OP_min1/1 -> Switch2/3
  Constant2/1 -> Switch2/2
  Switch2/1 -> ctrl/1

== system ACDCMG_woPV/Grid Bi-directional Converter 1.1 300 (DC) // 150 V (AC) P_nom 3kW2/Control of Inverter/MI Controller/Subsystem ==
  sin_cos : Inport  PortDimensions=2
  Demux : Demux  Outputs=2
      settings: DisplayOption=none
  Fcn2 : Fcn  Expr=1*u[1]
  Fcn4 : Fcn  Expr=1*u[3]
  Fcn5 : Fcn  Expr=1*u[5]
  K1 : Constant  Value=0.5
  K2 : Constant  Value=sqrt(3)/2
  Mux2 : Mux  Inputs=6
  Product{,1..3} (4 alike) : Product  InputSameDT=on  SaturateOnIntegerOverflow=on  OutDataTypeStr=Inherit: Same as first input
  Sum : Sum  Inputs=--  InputSameDT=on  SaturateOnIntegerOverflow=on  OutDataTypeStr=Inherit: Same as first input
  Sum1 : Sum  Inputs=-+  InputSameDT=on  SaturateOnIntegerOverflow=on  OutDataTypeStr=Inherit: Same as first input
  Sum2 : Sum  Inputs=--  InputSameDT=on  SaturateOnIntegerOverflow=on  OutDataTypeStr=Inherit: Same as first input
  Sum3 : Sum  Inputs=--  InputSameDT=on  SaturateOnIntegerOverflow=on  OutDataTypeStr=Inherit: Same as first input
  Va : Outport  VectorParamsAs1DForOutWhenUnconnected=off
  Vb : Outport  Port=2  VectorParamsAs1DForOutWhenUnconnected=off
  Vc : Outport  Port=3  VectorParamsAs1DForOutWhenUnconnected=off
  wires:
  sin_cos/1 -> Demux/1
  Demux/1 -> Product/1, Product2/1, Sum2/2, Mux2/1  "sin(wt)"
  Product/1 -> Sum/1
  Product1/1 -> Sum/2
  Product3/1 -> Sum1/1
  Product2/1 -> Sum1/2
  Sum3/1 -> Mux2/6  "cos(wt+2pi/3)"
  Sum2/1 -> Mux2/5  "sin(wt+2pi/3)"
  K1/1 -> Product/2, Product3/2
  K2/1 -> Product1/2, Product2/2
  Sum/1 -> Mux2/3, Sum2/1  "sin(wt-2pi/3)"
  Sum1/1 -> Mux2/4, Sum3/1  "cos(wt-2pi/3)"
  Demux/2 -> Sum3/2, Product3/1, Product1/1, Mux2/2  "cos(wt)"
  Mux2/1 -> Fcn2/1, Fcn4/1, Fcn5/1
  Fcn2/1 -> Va/1
  Fcn4/1 -> Vb/1
  Fcn5/1 -> Vc/1

== system ACDCMG_woPV/Grid Bi-directional Converter 1.1 300 (DC) // 150 V (AC) P_nom 3kW2/Control of Inverter/MI Controller/Subsystem1 ==
  note: AC to DC
  note: DC to AC
  Constant1 : Constant  Value=max_min
  Constant2 : Constant  Value=2*pi
  Deg->Rad : Gain  Gain=pi/180  SaturateOnIntegerOverflow=on  OutDataTypeStr=Inherit: Same as input  ParamDataTypeStr=Inherit: Same as input
  Freq1 : Constant  Value=Fnom
  Freq2 : Constant  Value=2*pi
  Math Function : Math  Operator=mod  SignedPower=on
  Mux5 : Mux  Inputs=2
  OP_max1 : Constant  Value=0
  OP_min1 : Constant  Value=228
  Product7 : Product  Inputs=***  InputSameDT=on  SaturateOnIntegerOverflow=on  OutDataTypeStr=Inherit: Same as first input
  Sum : Sum  InputSameDT=on  SaturateOnIntegerOverflow=on  OutDataTypeStr=Inherit: Same as first input
  Switch2 : Switch  Criteria=u2 > Threshold  SaturateOnIntegerOverflow=off  InputSameDT=off
  Trigonometric Function : Trigonometry
  Trigonometric Function1 : Trigonometry  Operator=cos
  t : DigitalClock  SampleTime=Ts
  Frec : Outport  VectorParamsAs1DForOutWhenUnconnected=off
  sin_cos : Outport  Port=2  VectorParamsAs1DForOutWhenUnconnected=off
  wt : Outport  Port=3  VectorParamsAs1DForOutWhenUnconnected=off
  wires:
  Switch2/1 -> Deg->Rad/1
  Deg->Rad/1 -> Sum/2
  Freq1/1 -> Frec/1, Product7/1
  Trigonometric Function/1 -> Mux5/1
  Sum/1 -> Math Function/1
  Trigonometric Function1/1 -> Mux5/2
  Product7/1 -> Sum/1
  Freq2/1 -> Product7/3
  Constant2/1 -> Math Function/2
  t/1 -> Product7/2
  Math Function/1 -> wt/1, Trigonometric Function1/1, Trigonometric Function/1
  Mux5/1 -> sin_cos/1
  Constant1/1 -> Switch2/2
  OP_max1/1 -> Switch2/1
  OP_min1/1 -> Switch2/3

== system ACDCMG_woPV/Grid Bi-directional Converter 1.2 300 (DC) // 150 V (AC) P_nom 3kW/Control of Inverter/MI Controller/Subsystem ==
  sin_cos : Inport  PortDimensions=2
  Demux : Demux  Outputs=2
      settings: DisplayOption=none
  Fcn2 : Fcn  Expr=1*u[1]
  Fcn4 : Fcn  Expr=1*u[3]
  Fcn5 : Fcn  Expr=1*u[5]
  K1 : Constant  Value=0.5
  K2 : Constant  Value=sqrt(3)/2
  Mux2 : Mux  Inputs=6
  Product{,1..3} (4 alike) : Product  InputSameDT=on  SaturateOnIntegerOverflow=on  OutDataTypeStr=Inherit: Same as first input
  Sum : Sum  Inputs=--  InputSameDT=on  SaturateOnIntegerOverflow=on  OutDataTypeStr=Inherit: Same as first input
  Sum1 : Sum  Inputs=-+  InputSameDT=on  SaturateOnIntegerOverflow=on  OutDataTypeStr=Inherit: Same as first input
  Sum2 : Sum  Inputs=--  InputSameDT=on  SaturateOnIntegerOverflow=on  OutDataTypeStr=Inherit: Same as first input
  Sum3 : Sum  Inputs=--  InputSameDT=on  SaturateOnIntegerOverflow=on  OutDataTypeStr=Inherit: Same as first input
  Va : Outport  VectorParamsAs1DForOutWhenUnconnected=off
  Vb : Outport  Port=2  VectorParamsAs1DForOutWhenUnconnected=off
  Vc : Outport  Port=3  VectorParamsAs1DForOutWhenUnconnected=off
  wires:
  sin_cos/1 -> Demux/1
  Demux/1 -> Product/1, Product2/1, Sum2/2, Mux2/1  "sin(wt)"
  Product/1 -> Sum/1
  Product1/1 -> Sum/2
  Product3/1 -> Sum1/1
  Product2/1 -> Sum1/2
  Sum3/1 -> Mux2/6  "cos(wt+2pi/3)"
  Sum2/1 -> Mux2/5  "sin(wt+2pi/3)"
  K1/1 -> Product/2, Product3/2
  K2/1 -> Product1/2, Product2/2
  Sum/1 -> Mux2/3, Sum2/1  "sin(wt-2pi/3)"
  Sum1/1 -> Mux2/4, Sum3/1  "cos(wt-2pi/3)"
  Demux/2 -> Sum3/2, Product3/1, Product1/1, Mux2/2  "cos(wt)"
  Mux2/1 -> Fcn2/1, Fcn4/1, Fcn5/1
  Fcn2/1 -> Va/1
  Fcn4/1 -> Vb/1
  Fcn5/1 -> Vc/1

== system ACDCMG_woPV/Grid Bi-directional Converter 1.2 300 (DC) // 150 V (AC) P_nom 3kW/Control of Inverter/MI Controller/Subsystem1 ==
  CD to AC : Constant  Value=0
  Constant2 : Constant  Value=2*pi
  Deg->Rad : Gain  Gain=pi/180  SaturateOnIntegerOverflow=on  OutDataTypeStr=Inherit: Same as input  ParamDataTypeStr=Inherit: Same as input
  Freq1 : Constant  Value=Fnom
  Freq2 : Constant  Value=2*pi
  Math Function : Math  Operator=mod  SignedPower=on
  Mux5 : Mux  Inputs=2
  Product7 : Product  Inputs=***  InputSameDT=on  SaturateOnIntegerOverflow=on  OutDataTypeStr=Inherit: Same as first input
  Sum : Sum  InputSameDT=on  SaturateOnIntegerOverflow=on  OutDataTypeStr=Inherit: Same as first input
  Trigonometric Function : Trigonometry
  Trigonometric Function1 : Trigonometry  Operator=cos
  t : DigitalClock  SampleTime=Ts
  Frec : Outport  VectorParamsAs1DForOutWhenUnconnected=off
  sin_cos : Outport  Port=2  VectorParamsAs1DForOutWhenUnconnected=off
  wt : Outport  Port=3  VectorParamsAs1DForOutWhenUnconnected=off
  wires:
  CD to AC/1 -> Deg->Rad/1
  Deg->Rad/1 -> Sum/2
  Freq1/1 -> Frec/1, Product7/1
  Trigonometric Function/1 -> Mux5/1
  Sum/1 -> Math Function/1
  Trigonometric Function1/1 -> Mux5/2
  Product7/1 -> Sum/1
  Freq2/1 -> Product7/3
  Constant2/1 -> Math Function/2
  t/1 -> Product7/2
  Math Function/1 -> wt/1, Trigonometric Function1/1, Trigonometric Function/1
  Mux5/1 -> sin_cos/1
